simulink model "Correlation_Stream_Ex2"  (R2024a)
settings: Solver=VariableStepAuto  StartTime=0.0  StopTime=2048/100e6  RelTol=1e-3
undefined symbols (not defined in the file): S, vsva2197, xcvc1902
libraries: dspstat3 x2, visionstatistics x1, aieDSP x1, aieUtilities x1, vmcUtilities x1
settings Model: Creator=sdegala  LastModifiedBy=sdegala
settings ModelReferenceCC: EnableRefExpFcnMdlSchedulingChecks=on
settings RTWCC: GPUComputeCapability=3.5
settings ConfigComp: CovBoundaryAbsTol=1.0e-5

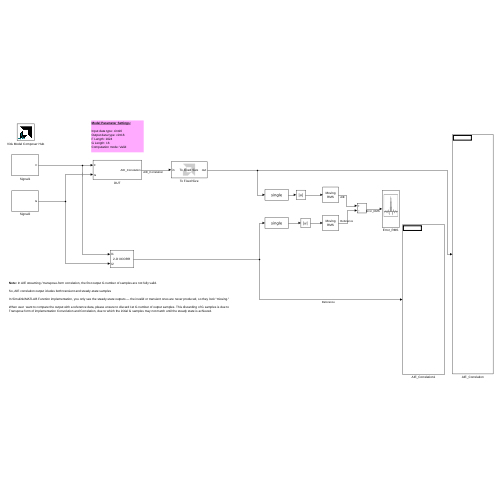
[thumbnail: Simulink's stored preview of the top-level diagram]
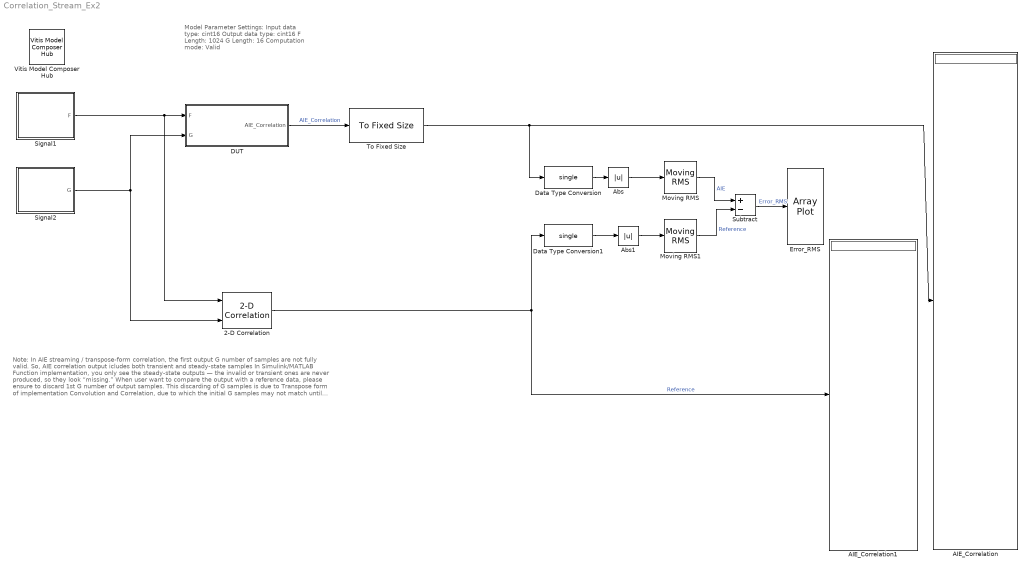
== system Correlation_Stream_Ex2 ==
  note: Note: In AIE streaming / transpose-form correlation, the first output G number of samples are not fully valid.
      |
      | So, AIE correlation output icludes both transient and steady-state samples
      |
      | In Simulink/MATLAB Function implementation, you only see the steady-state outputs — the invalid or transient ones are never produced, so they look “missing.”
      |
      | When user want to compare the output with a reference data, please ensure to discard 1st G number of output samples. This discarding of G samples is due to Transpose form of implementation Convolution and Correlation, due to which the initial G samples may not match until the steady state is achieved.
  note: Model Parameter Settings:
      |
      | Input data type: cint16
      | Output data type: cint16
      | F Length: 1024
      | G Length: 16
      | Computation mode: Valid
  2-D Correlation : visionstatistics/2-D Correlation  outSize=Valid  normalize=off  roundingMode=Floor  overflowMode=off
  AIE_Correlation : Display
  AIE_Correlation1 : Display
  Abs : Abs  SaturateOnIntegerOverflow=off
  Abs1 : Abs  SaturateOnIntegerOverflow=off
  DUT : Subsystem
  Data Type Conversion : DataTypeConversion  OutDataTypeStr=single  SaturateOnIntegerOverflow=off  RndMeth=Floor
  Data Type Conversion1 : DataTypeConversion  OutDataTypeStr=single  SaturateOnIntegerOverflow=off  RndMeth=Floor
  Error_RMS : ArrayPlot  WindowPosition=[1.000000,1.000000,1920.000000,1127.000000,]  Visible=on  ScopeFrameLocation=window  AxesScaling=Manual  YLimits=[-1 20]  ShowLegend=on
  Moving RMS : dspstat3/Moving RMS  Method=Sliding window  ForgettingFactorPort=off  SpecifyWindowLength=off  WindowLength=4  OverlapLength=3  AllowArbitraryInputLength=off  ForgettingFactor=0.9  SimulateUsing=Interpreted execution
  Moving RMS1 : dspstat3/Moving RMS  Method=Sliding window  ForgettingFactorPort=off  SpecifyWindowLength=off  WindowLength=4  OverlapLength=3  AllowArbitraryInputLength=off  ForgettingFactor=0.9  SimulateUsing=Interpreted execution
  Signal1 : Subsystem
  Signal2 : Subsystem
  Subtract : Sum  Inputs=+-
  To Fixed Size : aieUtilities/To Fixed Size  Mode=Stop simulation when input variable-size signal is not full  OutputSize=Inherit: Same as input  CopyMethod=Buffer samples to form output  HasStatusOutput=on
  Vitis Model Composer Hub : vmcUtilities/Vitis Model Composer Hub  Tag=genX  CodeGeneration=off  StartColumn=1  NumberOfColumns=1  TargetDirectory=./code  exportDesign=off  analyzeDesign=off  validateDesignOnHw=off  ExportType=AI Engines  IpVendor=xilinx.com  IpLibrary=hls  IpVersion=1.0  IpHWLanguage=Verilog  AieCompilerOptions={}  AieSimulatorOptions={}  CreateTestbench=off  TestbenchStackSize=10  RunRtlSim=off  RunCSim=off  RunAieSim=off  AieSimTimeout=50000  RunAieSimProfiling=off  LaunchVitisAnalyzer=off  PlotOutput=off  RunX86Sim=off  X86SimTimeout=10  GenHwImage=off  GenLibadfXo=off  GenHwValidationCode=off  PlatformType=Not Specified  HwSystemType=Baremetal  HwValidationTarget=hw  ProjDevice=xcvc1902-vsva2197-1LP-e-S  ProjDevicePart=xcvc1902-vsva2197-1LP-e-S  AIEType=AIE  SamplePeriod=-1  ClockFrequency=200  DataPathParallelism=1  xilinxfamily=versalaicore  part=xcvc1902  speed=-1LP-e-S  package=vsva2197  directory=./netlist  testbench=off  incr_netlist=off  synthesis_tool=Vivado  clock_wrapper=Clock Enables  dbl_ovrd=According to Block Masks  dcm_input_clock_period=10  sysclk_period=10  simulink_period=1  eval_field=0  LogFileName=''  NThreads=4
  wires:
  DUT/1(AIE_Correlation) -> To Fixed Size/1  "AIE_Correlation"
  Signal1/1(F) -> 2-D Correlation/1, DUT/1(F)
  Moving RMS/1 -> Subtract/1  "AIE"
  Moving RMS1/1 -> Subtract/2  "Reference"
  Data Type Conversion1/1 -> Abs1/1
  Data Type Conversion/1 -> Abs/1
  Abs/1 -> Moving RMS/1
  Abs1/1 -> Moving RMS1/1
  To Fixed Size/1 -> Data Type Conversion/1, AIE_Correlation/1
  Signal2/1(G) -> 2-D Correlation/2, DUT/2(G)
  2-D Correlation/1 -> Data Type Conversion1/1, AIE_Correlation1/1  "Reference"
  Subtract/1 -> Error_RMS/1  "Error_RMS"

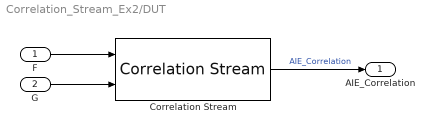
== system Correlation_Stream_Ex2/DUT ==
  F : Inport
  G : Inport  Port=2
  Correlation Stream : aieDSP/Correlation Stream  AIE_VARIANT=1  api=1  data_type_f=cint16  data_type_g=cint16  data_type_out=cint16  function_type=0  compute_mode=Valid  f_sample_size=1024  g_sample_size=16  USE_RTP_VECTOR_LENGTHS=off  num_frames=1  shift_output=0  rnd_mode=Floor  sat_mode=None  no_of_kernels=1  casc_length=1  blockJsonConstraints=[]  blockJsonConstraintsInternal=[]  spec=vmc_stream_corr.json  SerializedMaskParamNames=[]  SerializedMaskParamValues=[]  SerializedMaskParamVisibilities=[]  block_type=Correlation Stream  SerializedMaskParamDataypes=uint|uint|typename|typename|typename|uint|uint|uint|uint|uint|uint|uint|uint|uint|uint|uint  SerializedMaskParamEnumStrArr=0|0|0|0|0|0|Full,Same,Valid|0|0|0|0|0|Floor,Ceiling,Round to positive infinity,Round to negative infinity,Round symmetrical to infinity,Round symmetrical to zero,Round convergent to even,Round convergent to odd|None,Saturate,Symmetric|0|0  SerializedMaskParamEnumValArr=0|0|0|0|0|0|0,1,2|0|0|0|0|0|0,1,2,3,4,5,6,7|0,1,3|0|0  SerializedMaskParamVectorArr=0|0|0|0|0|0|0|0|0|0|0|0|0|0|0|0  SerializedMaskParamKeys=AIE_VARIANT|TP_API|TT_DATA_F|TT_DATA_G|TT_DATA_OUT|TP_FUNCT_TYPE|TP_COMPUTE_MODE|TP_F_LEN|TP_G_LEN|TP_USE_RTP_VECTOR_LENGTHS|TP_NUM_FRAMES|TP_SHIFT|TP_RND|TP_SAT|TP_PHASES|TP_CASC_LEN
  AIE_Correlation : Outport
  wires:
  F/1 -> Correlation Stream/1
  G/1 -> Correlation Stream/2
  Correlation Stream/1 -> AIE_Correlation/1  "AIE_Correlation"

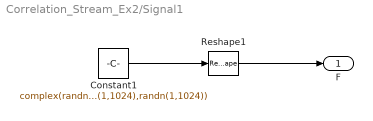
== system Correlation_Stream_Ex2/Signal1 ==
  Constant1 : Constant  Value=complex(randn(1,1024),randn(1,1024))  OutDataTypeStr=int16  SampleTime=1/100e6
  Reshape1 : Reshape
  F : Outport
  wires:
  Reshape1/1 -> F/1
  Constant1/1 -> Reshape1/1

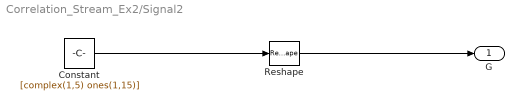
== system Correlation_Stream_Ex2/Signal2 ==
  Constant : Constant  Value=[complex(1,5) ones(1,15)]  OutDataTypeStr=int16  SampleTime=1/100e6
  Reshape : Reshape
  G : Outport
  wires:
  Reshape/1 -> G/1
  Constant/1 -> Reshape/1
